simulink model "pid_test_plant"  (R2016a)
settings: Solver=VariableStepAuto  StartTime=0.0  StopTime=500.0  RelTol=1e-3
settings Model: Creator=Matias  LastModifiedBy=Matias

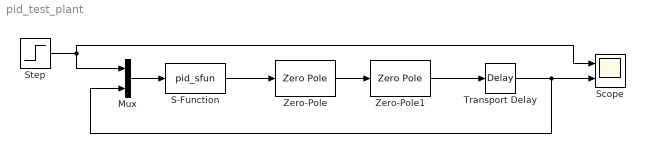
== system pid_test_plant ==
  Mux : Mux  Inputs=2
  S-Function : S-Function  FunctionName=pid_sfun  Parameters=3.0, 0.01, 1.0, 2.5, 1/50.0  SFunctionDeploymentMode=off  EnableBusSupport=off
  Scope : Scope  NumInputPorts=2
  Step : Step  SampleTime=0
  Transport Delay : TransportDelay  DelayTime=5
  Zero-Pole : ZeroPole  Zeros=[]  Poles=[-1/10]  Gain=[1/10]
  Zero-Pole1 : ZeroPole  Zeros=[]  Poles=[-1/60]  Gain=[1/60]
  wires:
  Mux/1 -> S-Function/1
  Step/1 -> Mux/1, Scope/1
  Zero-Pole/1 -> Zero-Pole1/1
  Zero-Pole1/1 -> Transport Delay/1
  Transport Delay/1 -> Mux/2, Scope/2
  S-Function/1 -> Zero-Pole/1
